simulink model "Comparação PD x Avanço - SimulinkArquivo"  (R2019a)
settings: Solver=VariableStepAuto  StartTime=0.0  StopTime=6  RelTol=1e-3
libraries: simulink x2
settings Model: Creator=rcard  LastModifiedBy=rcard

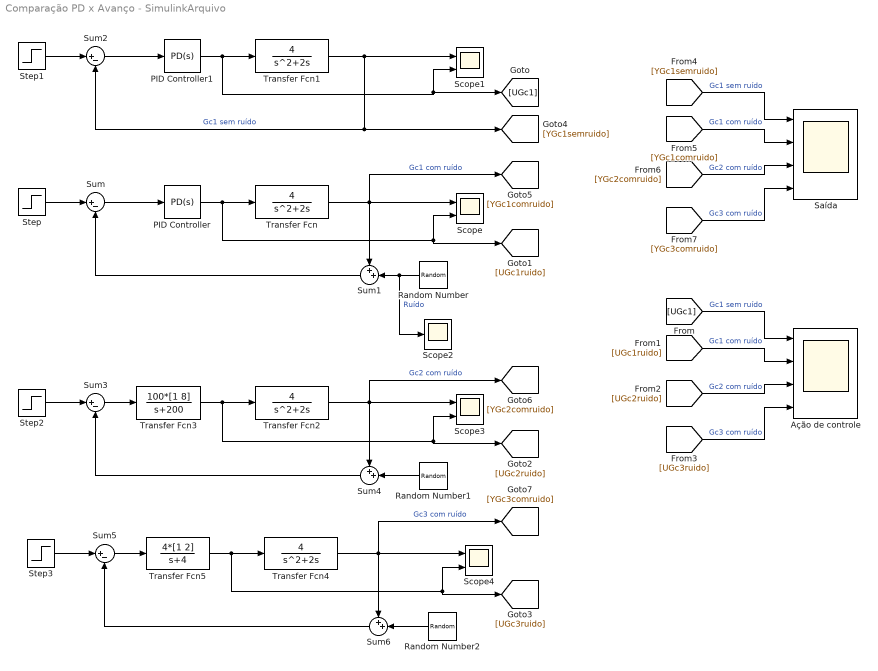
== system Comparação PD x Avanço - SimulinkArquivo ==
  Ação de controle : Scope  NumInputPorts=4
  PID Controller : simulink/Continuous/PID Controller  Controller=PD  Form=Ideal  TimeDomain=Continuous-time  SampleTime=-1  IntegratorMethod=Forward Euler  FilterMethod=Forward Euler  ControllerParametersSource=internal  P=4  I=1  D=0.125  UseFilter=on  N=10000  TunerSelectOption=Transfer Function Based (PID Tuner App)  InitialConditionSource=internal  InitialConditionForIntegrator=0  InitialConditionForFilter=0  DifferentiatorICPrevScaledInput=0  ExternalReset=none  TrackingMode=off  Kt=1  LimitOutput=off  UpperSaturationLimit=inf  LowerSaturationLimit=-inf  LinearizeAsGain=on  AntiWindupMode=none  Kb=1  POutMin=[]  POutMax=[]  IOutMin=[]  IOutMax=[]  DOutMin=[]  DOutMax=[]  NOutMin=[]  NOutMax=[]  SumOutMin=[]  SumOutMax=[]  SaturationOutMin=[]  SaturationOutMax=[]  PParamMin=[]  PParamMax=[]  IParamMin=[]  IParamMax=[]  DParamMin=[]  DParamMax=[]  NParamMin=[]  NParamMax=[]  KbParamMin=[]  KbParamMax=[]  KtParamMin=[]  KtParamMax=[]  KbOutMin=[]  KbOutMax=[]  KtOutMin=[]  KtOutMax=[]  IntegratorOutMin=[]  IntegratorOutMax=[]  FilterOutMin=[]  FilterOutMax=[]  SumI1OutMin=[]  SumI1OutMax=[]  SumI2OutMin=[]  SumI2OutMax=[]  SumI3OutMin=[]  SumI3OutMax=[]  SumI4OutMin=[]  SumI4OutMax=[]  SumDOutMin=[]  SumDOutMax=[]  DifferentiatorOutMin=[]  DifferentiatorOutMax=[]  FilterDiffOutCoefMin=[]  FilterDiffOutCoefMax=[]  ReciprocalOutMin=[]  ReciprocalOutMax=[]  SumDenOutMin=[]  SumDenOutMax=[]  SumNumOutMin=[]  SumNumOutMax=[]  DivideOutMin=[]  DivideOutMax=[]  IntegratorContinuousStateAttributes=''  IntegratorStateMustResolveToSignalObject=off  IntegratorRTWStateStorageClass=Auto  FilterContinuousStateAttributes=''  FilterStateMustResolveToSignalObject=off  FilterRTWStateStorageClass=Auto  ParallelPVariant=Passthrough  IdealPVariant=InternalParameters  IVariant=Disabled  DVariant=InternalParameters  IntegratorVariant=Disabled  SatVariant=Disabled  AWVariant=Disabled  PCopyVariant=Disabled  TRVariant=Disabled  FdbkBlocksVariant=Forward  IdealPFdbkVariant=Disabled  SatFdbkVariant=Disabled  DerivativeFilterVariant=ContFilter  NVariant=InternalParameters  NCopyVariant=Disabled  FilterICVariant=InternalICsFilter  IntegratorICVariant=Disabled  ExternalResetVariant=Disabled  TRSumVariant=Passthrough  SumFdbkVariant=Disabled  SumVariant=Sum_PD
  PID Controller1 : simulink/Continuous/PID Controller  Controller=PD  Form=Ideal  TimeDomain=Continuous-time  SampleTime=-1  IntegratorMethod=Forward Euler  FilterMethod=Forward Euler  ControllerParametersSource=internal  P=4  I=1  D=0.125  UseFilter=on  N=10000  TunerSelectOption=Transfer Function Based (PID Tuner App)  InitialConditionSource=internal  InitialConditionForIntegrator=0  InitialConditionForFilter=0  DifferentiatorICPrevScaledInput=0  ExternalReset=none  TrackingMode=off  Kt=1  LimitOutput=off  UpperSaturationLimit=inf  LowerSaturationLimit=-inf  LinearizeAsGain=on  AntiWindupMode=none  Kb=1  POutMin=[]  POutMax=[]  IOutMin=[]  IOutMax=[]  DOutMin=[]  DOutMax=[]  NOutMin=[]  NOutMax=[]  SumOutMin=[]  SumOutMax=[]  SaturationOutMin=[]  SaturationOutMax=[]  PParamMin=[]  PParamMax=[]  IParamMin=[]  IParamMax=[]  DParamMin=[]  DParamMax=[]  NParamMin=[]  NParamMax=[]  KbParamMin=[]  KbParamMax=[]  KtParamMin=[]  KtParamMax=[]  KbOutMin=[]  KbOutMax=[]  KtOutMin=[]  KtOutMax=[]  IntegratorOutMin=[]  IntegratorOutMax=[]  FilterOutMin=[]  FilterOutMax=[]  SumI1OutMin=[]  SumI1OutMax=[]  SumI2OutMin=[]  SumI2OutMax=[]  SumI3OutMin=[]  SumI3OutMax=[]  SumI4OutMin=[]  SumI4OutMax=[]  SumDOutMin=[]  SumDOutMax=[]  DifferentiatorOutMin=[]  DifferentiatorOutMax=[]  FilterDiffOutCoefMin=[]  FilterDiffOutCoefMax=[]  ReciprocalOutMin=[]  ReciprocalOutMax=[]  SumDenOutMin=[]  SumDenOutMax=[]  SumNumOutMin=[]  SumNumOutMax=[]  DivideOutMin=[]  DivideOutMax=[]  IntegratorContinuousStateAttributes=''  IntegratorStateMustResolveToSignalObject=off  IntegratorRTWStateStorageClass=Auto  FilterContinuousStateAttributes=''  FilterStateMustResolveToSignalObject=off  FilterRTWStateStorageClass=Auto  ParallelPVariant=Passthrough  IdealPVariant=InternalParameters  IVariant=Disabled  DVariant=InternalParameters  IntegratorVariant=Disabled  SatVariant=Disabled  AWVariant=Disabled  PCopyVariant=Disabled  TRVariant=Disabled  FdbkBlocksVariant=Forward  IdealPFdbkVariant=Disabled  SatFdbkVariant=Disabled  DerivativeFilterVariant=ContFilter  NVariant=InternalParameters  NCopyVariant=Disabled  FilterICVariant=InternalICsFilter  IntegratorICVariant=Disabled  ExternalResetVariant=Disabled  TRSumVariant=Passthrough  SumFdbkVariant=Disabled  SumVariant=Sum_PD
  Random Number : RandomNumber  Variance=0.25^2  SampleTime=0.001
  Random Number1 : RandomNumber  Variance=0.25^2  SampleTime=0.001
  Random Number2 : RandomNumber  Variance=0.25^2  SampleTime=0.001
  Saída : Scope  NumInputPorts=4
  Scope{,1,3..4} (4 alike) : Scope  NumInputPorts=2
  Scope2 : Scope
  Step{,1..3} (4 alike) : Step  Time=0  SampleTime=0
  Sum{,2..3,5} (4 alike) : Sum  Inputs=|+-
  Sum1 : Sum  Inputs=++|
  Sum4 : Sum  Inputs=++|
  Sum6 : Sum  Inputs=++|
  Transfer Fcn{,1..2,4} (4 alike) : TransferFcn  Numerator=[4]  Denominator=[1 2 0]
  Transfer Fcn3 : TransferFcn  Numerator=100*[1 8]  Denominator=[1 200]
  Transfer Fcn5 : TransferFcn  Numerator=4*[1 2]  Denominator=[1 4]
  wires:
  Step/1 -> Sum/1
  Sum/1 -> PID Controller/1
  PID Controller/1 -> [UGc1ruido], Scope/2, Transfer Fcn/1
  Sum1/1 -> Sum/2
  Transfer Fcn/1 -> [YGc1comruido], Sum1/1, Scope/1  "Gc1 com ruído"
  Random Number/1 -> Scope2/1, Sum1/2  "Ruído"
  PID Controller1/1 -> [UGc1], Scope1/2, Transfer Fcn1/1
  Transfer Fcn1/1 -> [YGc1semruido], Sum2/2, Scope1/1  "Gc1 sem ruído"
  Step1/1 -> Sum2/1
  Sum2/1 -> PID Controller1/1
  Transfer Fcn3/1 -> [UGc2ruido], Scope3/2, Transfer Fcn2/1
  Transfer Fcn2/1 -> [YGc2comruido], Sum4/1, Scope3/1  "Gc2 com ruído"
  Random Number1/1 -> Sum4/2
  Sum4/1 -> Sum3/2
  Step2/1 -> Sum3/1
  Sum3/1 -> Transfer Fcn3/1
  Transfer Fcn5/1 -> [UGc3ruido], Scope4/2, Transfer Fcn4/1
  Step3/1 -> Sum5/1
  Transfer Fcn4/1 -> [YGc3comruido], Sum6/1, Scope4/1  "Gc3 com ruído"
  Random Number2/1 -> Sum6/2
  Sum5/1 -> Transfer Fcn5/1
  Sum6/1 -> Sum5/2
  [UGc1] -> Ação de controle/1  "Gc1 sem ruído"
  [UGc1ruido] -> Ação de controle/2  "Gc1 com ruído"
  [UGc2ruido] -> Ação de controle/3  "Gc2 com ruído"
  [UGc3ruido] -> Ação de controle/4  "Gc3 com ruído"
  [YGc2comruido] -> Saída/3  "Gc2 com ruído"
  [YGc3comruido] -> Saída/4  "Gc3 com ruído"
  [YGc1semruido] -> Saída/1  "Gc1 sem ruído"
  [YGc1comruido] -> Saída/2  "Gc1 com ruído"
